simulink model "ZT_VehCtrl_18B"  (R2018b)
settings: Solver=FixedStepAuto  StartTime=0.0  StopTime=inf  FixedStep=0.005  RelTol=1e-3
InitFcn:
  | mbd_mpc_consistency_checks(bdroot(gcs));
undefined symbols (not defined in the file): ANG_DEAD, BMS_NormalPwr, BrkPrsByBrkPct_TB_X, BrkPrsByBrkPct_TB_Y, DELAY_DISCHARGE, DELAY_RCUOFF, DRV_BACKWARD, DRV_BRAKE, DRV_FORWARD, DRV_NEUTRAL, DRV_PARK, DRV_UNPARK, DRV_ZEROTURN, EPB_LOCK, EPB_UNLOCK, ExtraLoadPwr, FanOff, fifo_0_vect, fifo_1_vect, HiFanReq, HV_finished, HV_No_Active, HV_POWER_OFF, HV_POWER_ON, HVDown, HVON, KaTLS_v_DrgUp_X_VehSpd, KeFTM_s_Way1OffDlyTime, KeFTM_TK_Way1CoolLv2OffBatTemp, KeFTM_TK_Way1CoolLv2OffMtrTemp, KeFTM_TK_Way1CoolLv2OnBatTemp, KeFTM_TK_Way1CoolLv2OnMtrTemp, KeFTM_TK_Way1CoolLv3OffBatTemp, KeFTM_TK_Way1CoolLv3OffMtrTemp, KeFTM_TK_Way1CoolLv3OnBatTemp, KeFTM_TK_Way1CoolLv3OnMtrTemp, KeFTM_TK_Way1CoolLv4OffBatTemp, KeFTM_TK_Way1CoolLv4OffMtrTemp, KeFTM_TK_Way1CoolLv4OnBatTemp, KeFTM_TK_Way1CoolLv4OnMtrTemp, Kp1, Kp2, LowFanReq, LQFP, MtrPwrFactor_RCU, MtrPwrHighToMidThd, MtrPwrLowToMidThd, MtrPwrMidToHighThd, MtrPwrMidToLowThd, MtrTrqMax, PCT_DEAD, Precharge, PTO_1000, PTO_540, pts1_fifo_0_vect, pts1_fifo_1_vect, pts2_fifo_0_vect, pts2_fifo_1_vect, pts3_fifo_0_vect, pts3_fifo_1_vect ... (+24)
libraries: mbd_mpc574x_ec_toolbox x124, canmsglib x72, simulink x57
(part 5 of 11)

== system ZT_VehCtrl_18B/SigIn/CAN1/ACU1 ==
  ID : Inport
  Data : Inport  Port=2
  length : Inport  Port=3
  timestamp : Inport  Port=4
  Switch Case : SwitchCase  CaseConditions={hex2dec('0C08A79A')}  ShowDefaultCase=off
  UNPACK : Subsystem  TreatAsAtomicUnit=on
  Message : Outport
  wires:
  Switch Case/1 -> UNPACK/Action
  ID/1 -> UNPACK/1(ID), Switch Case/1
  Data/1 -> UNPACK/2(data)
  timestamp/1 -> UNPACK/4(timestamp)
  length/1 -> UNPACK/3(length)
  UNPACK/1(Message) -> Message/1

== system ZT_VehCtrl_18B/SigIn/CAN1/ACU2 ==
  ID : Inport
  Data : Inport  Port=2
  length : Inport  Port=3
  timestamp : Inport  Port=4
  Switch Case : SwitchCase  CaseConditions={hex2dec('0C09A79B')}  ShowDefaultCase=off
  UNPACK : Subsystem  TreatAsAtomicUnit=on
  Message : Outport
  wires:
  UNPACK/1(Message) -> Message/1
  length/1 -> UNPACK/3(length)
  timestamp/1 -> UNPACK/4(timestamp)
  Data/1 -> UNPACK/2(data)
  ID/1 -> Switch Case/1, UNPACK/1(ID)
  Switch Case/1 -> UNPACK/Action

== system ZT_VehCtrl_18B/SigIn/CAN1/ACU3 ==
  ID : Inport
  Data : Inport  Port=2
  length : Inport  Port=3
  timestamp : Inport  Port=4
  Switch Case : SwitchCase  CaseConditions={hex2dec('0C0AA79D')}  ShowDefaultCase=off
  UNPACK : Subsystem  TreatAsAtomicUnit=on
  Message : Outport
  wires:
  Switch Case/1 -> UNPACK/Action
  ID/1 -> UNPACK/1(ID), Switch Case/1
  Data/1 -> UNPACK/2(data)
  timestamp/1 -> UNPACK/4(timestamp)
  length/1 -> UNPACK/3(length)
  UNPACK/1(Message) -> Message/1

== system ZT_VehCtrl_18B/SigIn/CAN1/HVC1_LV ==
  ID : Inport
  Data : Inport  Port=2
  length : Inport  Port=3
  timestamp : Inport  Port=4
  Switch Case : SwitchCase  CaseConditions={hex2dec('180105A1')}  ShowDefaultCase=off
  UNPACK : Subsystem  TreatAsAtomicUnit=on
  Message : Outport
  wires:
  Switch Case/1 -> UNPACK/Action
  ID/1 -> UNPACK/1(ID), Switch Case/1
  Data/1 -> UNPACK/2(data)
  timestamp/1 -> UNPACK/4(timestamp)
  length/1 -> UNPACK/3(length)
  UNPACK/1(Message) -> Message/1

== system ZT_VehCtrl_18B/SigIn/CAN1/HVC3_Temp ==
  ID : Inport
  Data : Inport  Port=2
  length : Inport  Port=3
  timestamp : Inport  Port=4
  Switch Case : SwitchCase  CaseConditions={hex2dec('180305A1')}  ShowDefaultCase=off
  UNPACK : Subsystem  TreatAsAtomicUnit=on
  Message : Outport
  wires:
  UNPACK/1(Message) -> Message/1
  length/1 -> UNPACK/3(length)
  timestamp/1 -> UNPACK/4(timestamp)
  Data/1 -> UNPACK/2(data)
  ID/1 -> Switch Case/1, UNPACK/1(ID)
  Switch Case/1 -> UNPACK/Action

== system ZT_VehCtrl_18B/SigIn/CAN1/HVC4_RlySt ==
  ID : Inport
  Data : Inport  Port=2
  length : Inport  Port=3
  timestamp : Inport  Port=4
  Switch Case : SwitchCase  CaseConditions={hex2dec('180405A1')}  ShowDefaultCase=off
  UNPACK : Subsystem  TreatAsAtomicUnit=on
  Message : Outport
  wires:
  Switch Case/1 -> UNPACK/Action
  ID/1 -> UNPACK/1(ID), Switch Case/1
  Data/1 -> UNPACK/2(data)
  timestamp/1 -> UNPACK/4(timestamp)
  length/1 -> UNPACK/3(length)
  UNPACK/1(Message) -> Message/1

== system ZT_VehCtrl_18B/SigIn/CAN1/HVC7_HV1 ==
  ID : Inport
  Data : Inport  Port=2
  length : Inport  Port=3
  timestamp : Inport  Port=4
  Switch Case : SwitchCase  CaseConditions={hex2dec('180705A1')}  ShowDefaultCase=off
  UNPACK : Subsystem  TreatAsAtomicUnit=on
  Message : Outport
  wires:
  UNPACK/1(Message) -> Message/1
  length/1 -> UNPACK/3(length)
  timestamp/1 -> UNPACK/4(timestamp)
  Data/1 -> UNPACK/2(data)
  ID/1 -> Switch Case/1, UNPACK/1(ID)
  Switch Case/1 -> UNPACK/Action

== system ZT_VehCtrl_18B/SigIn/CAN1/ISG MCU STATUS 1 ==
  ID : Inport
  Data : Inport  Port=2
  length : Inport  Port=3
  timestamp : Inport  Port=4
  Switch Case : SwitchCase  CaseConditions={hex2dec('CFF0006')}  ShowDefaultCase=off
  UNPACK : Subsystem  TreatAsAtomicUnit=on
  Message : Outport
  wires:
  Switch Case/1 -> UNPACK/Action
  ID/1 -> UNPACK/1(ID), Switch Case/1
  Data/1 -> UNPACK/2(data)
  timestamp/1 -> UNPACK/4(timestamp)
  length/1 -> UNPACK/3(length)
  UNPACK/1(Message) -> Message/1

== system ZT_VehCtrl_18B/SigIn/CAN1/ISG MCU STATUS 2 ==
  ID : Inport
  Data : Inport  Port=2
  length : Inport  Port=3
  timestamp : Inport  Port=4
  Switch Case : SwitchCase  CaseConditions={hex2dec('CFF0106')}  ShowDefaultCase=off
  UNPACK : Subsystem  TreatAsAtomicUnit=on
  Message : Outport
  wires:
  UNPACK/1(Message) -> Message/1
  length/1 -> UNPACK/3(length)
  timestamp/1 -> UNPACK/4(timestamp)
  Data/1 -> UNPACK/2(data)
  ID/1 -> Switch Case/1, UNPACK/1(ID)
  Switch Case/1 -> UNPACK/Action

== system ZT_VehCtrl_18B/SigIn/CAN1/ISG MCU STATUS 3 ==
  ID : Inport
  Data : Inport  Port=2
  length : Inport  Port=3
  timestamp : Inport  Port=4
  Switch Case : SwitchCase  CaseConditions={hex2dec('CFF0206')}  ShowDefaultCase=off
  UNPACK : Subsystem  TreatAsAtomicUnit=on
  Message : Outport
  wires:
  Switch Case/1 -> UNPACK/Action
  ID/1 -> UNPACK/1(ID), Switch Case/1
  Data/1 -> UNPACK/2(data)
  timestamp/1 -> UNPACK/4(timestamp)
  length/1 -> UNPACK/3(length)
  UNPACK/1(Message) -> Message/1

== system ZT_VehCtrl_18B/SigIn/CAN1/MCU1Msg1 ==
  ID : Inport
  Data : Inport  Port=2
  length : Inport  Port=3
  timestamp : Inport  Port=4
  Switch Case : SwitchCase  CaseConditions={hex2dec('1836D0EF')}  ShowDefaultCase=off
  UNPACK : Subsystem  TreatAsAtomicUnit=on
  Message : Outport
  wires:
  UNPACK/1(Message) -> Message/1
  length/1 -> UNPACK/3(length)
  timestamp/1 -> UNPACK/4(timestamp)
  Data/1 -> UNPACK/2(data)
  ID/1 -> Switch Case/1, UNPACK/1(ID)
  Switch Case/1 -> UNPACK/Action

== system ZT_VehCtrl_18B/SigIn/CAN1/MCU1Msg2 ==
  ID : Inport
  Data : Inport  Port=2
  length : Inport  Port=3
  timestamp : Inport  Port=4
  Switch Case : SwitchCase  CaseConditions={hex2dec('1837D0EF')}  ShowDefaultCase=off
  UNPACK : Subsystem  TreatAsAtomicUnit=on
  Message : Outport
  wires:
  Switch Case/1 -> UNPACK/Action
  ID/1 -> UNPACK/1(ID), Switch Case/1
  Data/1 -> UNPACK/2(data)
  timestamp/1 -> UNPACK/4(timestamp)
  length/1 -> UNPACK/3(length)
  UNPACK/1(Message) -> Message/1

== system ZT_VehCtrl_18B/SigIn/CAN1/MCU1Msg3 ==
  ID : Inport
  Data : Inport  Port=2
  length : Inport  Port=3
  timestamp : Inport  Port=4
  Switch Case : SwitchCase  CaseConditions={hex2dec('1838D0EF')}  ShowDefaultCase=off
  UNPACK : Subsystem  TreatAsAtomicUnit=on
  Message : Outport
  wires:
  UNPACK/1(Message) -> Message/1
  length/1 -> UNPACK/3(length)
  timestamp/1 -> UNPACK/4(timestamp)
  Data/1 -> UNPACK/2(data)
  ID/1 -> Switch Case/1, UNPACK/1(ID)
  Switch Case/1 -> UNPACK/Action

== system ZT_VehCtrl_18B/SigIn/CAN1/MCU2Msg1 ==
  ID : Inport
  Data : Inport  Port=2
  length : Inport  Port=3
  timestamp : Inport  Port=4
  Switch Case : SwitchCase  CaseConditions={hex2dec('1836D0F1')}  ShowDefaultCase=off
  UNPACK : Subsystem  TreatAsAtomicUnit=on
  Message : Outport
  wires:
  Switch Case/1 -> UNPACK/Action
  ID/1 -> UNPACK/1(ID), Switch Case/1
  Data/1 -> UNPACK/2(data)
  timestamp/1 -> UNPACK/4(timestamp)
  length/1 -> UNPACK/3(length)
  UNPACK/1(Message) -> Message/1

== system ZT_VehCtrl_18B/SigIn/CAN1/MCU2Msg2 ==
  ID : Inport
  Data : Inport  Port=2
  length : Inport  Port=3
  timestamp : Inport  Port=4
  Switch Case : SwitchCase  CaseConditions={hex2dec('1837D0F1')}  ShowDefaultCase=off
  UNPACK : Subsystem  TreatAsAtomicUnit=on
  Message : Outport
  wires:
  UNPACK/1(Message) -> Message/1
  length/1 -> UNPACK/3(length)
  timestamp/1 -> UNPACK/4(timestamp)
  Data/1 -> UNPACK/2(data)
  ID/1 -> Switch Case/1, UNPACK/1(ID)
  Switch Case/1 -> UNPACK/Action

== system ZT_VehCtrl_18B/SigIn/CAN1/MCU2Msg3 ==
  ID : Inport
  Data : Inport  Port=2
  length : Inport  Port=3
  timestamp : Inport  Port=4
  Switch Case : SwitchCase  CaseConditions={hex2dec('1838D0F1')}  ShowDefaultCase=off
  UNPACK : Subsystem  TreatAsAtomicUnit=on
  Message : Outport
  wires:
  Switch Case/1 -> UNPACK/Action
  ID/1 -> UNPACK/1(ID), Switch Case/1
  Data/1 -> UNPACK/2(data)
  timestamp/1 -> UNPACK/4(timestamp)
  length/1 -> UNPACK/3(length)
  UNPACK/1(Message) -> Message/1

== system ZT_VehCtrl_18B/SigIn/CAN1/PDU_RelaySts ==
  ID : Inport
  Data : Inport  Port=2
  length : Inport  Port=3
  timestamp : Inport  Port=4
  Switch Case : SwitchCase  CaseConditions={hex2dec('18FF2BC8')}  ShowDefaultCase=off
  UNPACK : Subsystem  TreatAsAtomicUnit=on
  Message : Outport
  wires:
  UNPACK/1(Message) -> Message/1
  length/1 -> UNPACK/3(length)
  timestamp/1 -> UNPACK/4(timestamp)
  Data/1 -> UNPACK/2(data)
  ID/1 -> Switch Case/1, UNPACK/1(ID)
  Switch Case/1 -> UNPACK/Action

== system ZT_VehCtrl_18B/SigIn/CAN1/TM MCU STATUS 1 ==
  ID : Inport
  Data : Inport  Port=2
  length : Inport  Port=3
  timestamp : Inport  Port=4
  Switch Case : SwitchCase  CaseConditions={hex2dec('CFF0005')}  ShowDefaultCase=off
  UNPACK : Subsystem  TreatAsAtomicUnit=on
  Message : Outport
  wires:
  UNPACK/1(Message) -> Message/1
  length/1 -> UNPACK/3(length)
  timestamp/1 -> UNPACK/4(timestamp)
  Data/1 -> UNPACK/2(data)
  ID/1 -> Switch Case/1, UNPACK/1(ID)
  Switch Case/1 -> UNPACK/Action

== system ZT_VehCtrl_18B/SigIn/CAN1/TM MCU STATUS 2 ==
  ID : Inport
  Data : Inport  Port=2
  length : Inport  Port=3
  timestamp : Inport  Port=4
  Switch Case : SwitchCase  CaseConditions={hex2dec('CFF0105')}  ShowDefaultCase=off
  UNPACK : Subsystem  TreatAsAtomicUnit=on
  Message : Outport
  wires:
  Switch Case/1 -> UNPACK/Action
  ID/1 -> UNPACK/1(ID), Switch Case/1
  Data/1 -> UNPACK/2(data)
  timestamp/1 -> UNPACK/4(timestamp)
  length/1 -> UNPACK/3(length)
  UNPACK/1(Message) -> Message/1

== system ZT_VehCtrl_18B/SigIn/CAN1/TM MCU STATUS 3 ==
  ID : Inport
  Data : Inport  Port=2
  length : Inport  Port=3
  timestamp : Inport  Port=4
  Switch Case : SwitchCase  CaseConditions={hex2dec('CFF0205')}  ShowDefaultCase=off
  UNPACK : Subsystem  TreatAsAtomicUnit=on
  Message : Outport
  wires:
  UNPACK/1(Message) -> Message/1
  length/1 -> UNPACK/3(length)
  timestamp/1 -> UNPACK/4(timestamp)
  Data/1 -> UNPACK/2(data)
  ID/1 -> Switch Case/1, UNPACK/1(ID)
  Switch Case/1 -> UNPACK/Action

== system ZT_VehCtrl_18B/SigIn/CAN1/TWV  ==
  ID : Inport
  Data : Inport  Port=2
  length : Inport  Port=3
  timestamp : Inport  Port=4
  Switch Case : SwitchCase  CaseConditions={hex2dec('18FF243B')}  ShowDefaultCase=off
  UNPACK : Subsystem  TreatAsAtomicUnit=on
  Message : Outport
  wires:
  Switch Case/1 -> UNPACK/Action
  ID/1 -> UNPACK/1(ID), Switch Case/1
  Data/1 -> UNPACK/2(data)
  timestamp/1 -> UNPACK/4(timestamp)
  length/1 -> UNPACK/3(length)
  UNPACK/1(Message) -> Message/1

== system ZT_VehCtrl_18B/SigIn/DI/DI_31_32_33_34 ==
  note: DI PWM PULLUP
  note: DI PWM PULLDOWN
  DI31 : mbd_mpc574x_ec_toolbox/GPIO Blocks/Digital_Input  gpio_pin=PTF0: [SIUL2_GPIO80 | General Purpose IO PF[0]]  pull_resistor=None
  DI32 : mbd_mpc574x_ec_toolbox/GPIO Blocks/Digital_Input  gpio_pin=PTD1: [SIUL2_GPIO49 | General Purpose IO PD[1]]  pull_resistor=None
  DI33 : mbd_mpc574x_ec_toolbox/GPIO Blocks/Digital_Input  gpio_pin=PTD2: [SIUL2_GPIO50 | General Purpose IO PD[2]]  pull_resistor=None
  DI34 : mbd_mpc574x_ec_toolbox/GPIO Blocks/Digital_Input  gpio_pin=PTC13: [SIUL2_GPIO45 | General Purpose IO PC[13]]  pull_resistor=None
  Data Store Write14 : DataStoreWrite  DataStoreName=DI31
  Data Store Write15 : DataStoreWrite  DataStoreName=DI32
  Data Store Write16 : DataStoreWrite  DataStoreName=DI33
  Data Store Write17 : DataStoreWrite  DataStoreName=DI34
  wires:
  DI34/1 -> Data Store Write17/1
  DI33/1 -> Data Store Write16/1
  DI32/1 -> Data Store Write15/1
  DI31/1 -> Data Store Write14/1

== system ZT_VehCtrl_18B/SigIn/PWM/PWM_PTS1 ==
  Add : Sum  Inputs=+-  AccumDataTypeStr=single
  Add1 : Sum  Inputs=+-  AccumDataTypeStr=single
  Data Store Memory : DataStoreMemory  DataStoreName=pts1_pwm_cnt  ReadBeforeWriteMsg=warning  WriteAfterWriteMsg=warning  WriteAfterReadMsg=warning  ShowAdditionalParam=off  OutDataTypeStr=uint8
  Data Store Memory2 : DataStoreMemory  DataStoreName=pts1_fifo_1_vect  ReadBeforeWriteMsg=warning  WriteAfterWriteMsg=warning  WriteAfterReadMsg=warning  InitialValue=[0 0 0 0 0 0 0 0]  ShowAdditionalParam=off  OutDataTypeStr=uint16
  Data Store Memory4 : DataStoreMemory  DataStoreName=pts1_fifo_0_vect  ReadBeforeWriteMsg=warning  WriteAfterWriteMsg=warning  WriteAfterReadMsg=warning  InitialValue=[0 0 0 0 0 0 0 0]  ShowAdditionalParam=off  OutDataTypeStr=uint16
  Data Store Read : DataStoreRead  DataStoreName=pts1_fifo_0_vect  DataStoreElements=pts1_fifo_0_vect(2)#pts1_fifo_0_vect(1)
  Data Store Read1 : DataStoreRead  DataStoreName=pts1_fifo_1_vect  DataStoreElements=pts1_fifo_1_vect(1)
  Data Store Read2 : DataStoreRead  DataStoreName=pts1_fifo_0_vect  DataStoreElements=pts1_fifo_0_vect(1)
  Data Store Write3 : DataStoreWrite  DataStoreName=pts1_fifo_0_vect
  Data Store Write5 : DataStoreWrite  DataStoreName=pts1_fifo_1_vect
  Divide : Product  Inputs=*/  OutDataTypeStr=single
  Divide1 : Product  Inputs=*//
  Freq_MC : Constant  Value=80000000  OutDataTypeStr=single
  Prescaler : Constant  Value=32  OutDataTypeStr=single
  Subsystem : Subsystem
  Subsystem_capture : Subsystem
  Terminator1 : Terminator
  Terminator2 : Terminator
  eTimer_ISR : mbd_mpc574x_ec_toolbox/Motor Control Blocks/eTIMER Blocks/eTimer_ISR_Handler  etimerModule=1  etimerInterrupt=Channel Interrupt  etimerChannel=2  etimerIsrPriority=14
      settings: SourceProductName=NXP Model-Based Design Toolbox for MPC57xx MCUs
  DC : Outport
  freq : Outport  Port=2
  wires:
  eTimer_ISR/2 -> Subsystem_capture/1(In1)
  Subsystem_capture/1(Out1) -> Terminator1/1
  Subsystem_capture/3(Out3) -> Terminator2/1
  Subsystem_capture/4(Out4) -> Data Store Write5/1
  Subsystem_capture/2(Out2) -> Data Store Write3/1
  eTimer_ISR/1 -> Subsystem_capture/Trigger
  Prescaler/1 -> Divide1/2
  Add/1 -> Divide/2, Divide1/3
  Data Store Read1/1 -> Add1/1
  Data Store Read/2 -> Add/2
  Freq_MC/1 -> Divide1/1
  Add1/1 -> Divide/1
  Data Store Read2/1 -> Add1/2
  Divide1/1 -> freq/1
  Data Store Read/1 -> Add/1
  Divide/1 -> Subsystem/1(In1)
  Subsystem/1(Out1) -> DC/1

== system ZT_VehCtrl_18B/SigIn/PWM/PWM_PTS2 ==
  Add : Sum  Inputs=+-  AccumDataTypeStr=single
  Add1 : Sum  Inputs=+-  AccumDataTypeStr=single
  Data Store Memory : DataStoreMemory  DataStoreName=pts2_pwm_cnt  ReadBeforeWriteMsg=warning  WriteAfterWriteMsg=warning  WriteAfterReadMsg=warning  ShowAdditionalParam=off  OutDataTypeStr=uint8
  Data Store Memory2 : DataStoreMemory  DataStoreName=pts2_fifo_1_vect  ReadBeforeWriteMsg=warning  WriteAfterWriteMsg=warning  WriteAfterReadMsg=warning  InitialValue=[0 0 0 0 0 0 0 0]  ShowAdditionalParam=off  OutDataTypeStr=uint16
  Data Store Memory4 : DataStoreMemory  DataStoreName=pts2_fifo_0_vect  ReadBeforeWriteMsg=warning  WriteAfterWriteMsg=warning  WriteAfterReadMsg=warning  InitialValue=[0 0 0 0 0 0 0 0]  ShowAdditionalParam=off  OutDataTypeStr=uint16
  Data Store Read : DataStoreRead  DataStoreName=pts2_fifo_0_vect  DataStoreElements=pts2_fifo_0_vect(2)#pts2_fifo_0_vect(1)
  Data Store Read1 : DataStoreRead  DataStoreName=pts2_fifo_1_vect  DataStoreElements=pts2_fifo_1_vect(1)
  Data Store Read2 : DataStoreRead  DataStoreName=pts2_fifo_0_vect  DataStoreElements=pts2_fifo_0_vect(1)
  Data Store Write3 : DataStoreWrite  DataStoreName=pts2_fifo_0_vect
  Data Store Write5 : DataStoreWrite  DataStoreName=pts2_fifo_1_vect
  Divide : Product  Inputs=*/  OutDataTypeStr=single
  Divide1 : Product  Inputs=*//
  Freq_MC : Constant  Value=80000000  OutDataTypeStr=single
  Prescaler : Constant  Value=32  OutDataTypeStr=single
  Subsystem : Subsystem
  Subsystem_capture : Subsystem
  Terminator1 : Terminator
  Terminator2 : Terminator
  eTimer_ISR : mbd_mpc574x_ec_toolbox/Motor Control Blocks/eTIMER Blocks/eTimer_ISR_Handler  etimerModule=1  etimerInterrupt=Channel Interrupt  etimerChannel=3  etimerIsrPriority=14
      settings: SourceProductName=NXP Model-Based Design Toolbox for MPC57xx MCUs
  DC : Outport
  freq : Outport  Port=2
  wires:
  Subsystem/1(Out1) -> DC/1
  Divide/1 -> Subsystem/1(In1)
  Data Store Read/1 -> Add/1
  Divide1/1 -> freq/1
  Data Store Read2/1 -> Add1/2
  Add1/1 -> Divide/1
  Freq_MC/1 -> Divide1/1
  Data Store Read/2 -> Add/2
  Data Store Read1/1 -> Add1/1
  Add/1 -> Divide1/3, Divide/2
  Prescaler/1 -> Divide1/2
  eTimer_ISR/1 -> Subsystem_capture/Trigger
  Subsystem_capture/2(Out2) -> Data Store Write3/1
  Subsystem_capture/4(Out4) -> Data Store Write5/1
  Subsystem_capture/3(Out3) -> Terminator2/1
  Subsystem_capture/1(Out1) -> Terminator1/1
  eTimer_ISR/2 -> Subsystem_capture/1(In1)

== system ZT_VehCtrl_18B/SigIn/PWM/PWM_PTS3 ==
  Add : Sum  Inputs=+-  AccumDataTypeStr=single
  Add1 : Sum  Inputs=+-  AccumDataTypeStr=single
  Data Store Memory : DataStoreMemory  DataStoreName=pts3_pwm_cnt  ReadBeforeWriteMsg=warning  WriteAfterWriteMsg=warning  WriteAfterReadMsg=warning  ShowAdditionalParam=off  OutDataTypeStr=uint8
  Data Store Memory2 : DataStoreMemory  DataStoreName=pts3_fifo_1_vect  ReadBeforeWriteMsg=warning  WriteAfterWriteMsg=warning  WriteAfterReadMsg=warning  InitialValue=[0 0 0 0 0 0 0 0]  ShowAdditionalParam=off  OutDataTypeStr=uint16
  Data Store Memory4 : DataStoreMemory  DataStoreName=pts3_fifo_0_vect  ReadBeforeWriteMsg=warning  WriteAfterWriteMsg=warning  WriteAfterReadMsg=warning  InitialValue=[0 0 0 0 0 0 0 0]  ShowAdditionalParam=off  OutDataTypeStr=uint16
  Data Store Read : DataStoreRead  DataStoreName=pts3_fifo_0_vect  DataStoreElements=pts3_fifo_0_vect(2)#pts3_fifo_0_vect(1)
  Data Store Read1 : DataStoreRead  DataStoreName=pts3_fifo_1_vect  DataStoreElements=pts3_fifo_1_vect(1)
  Data Store Read2 : DataStoreRead  DataStoreName=pts3_fifo_0_vect  DataStoreElements=pts3_fifo_0_vect(1)
  Data Store Write3 : DataStoreWrite  DataStoreName=pts3_fifo_0_vect
  Data Store Write5 : DataStoreWrite  DataStoreName=pts3_fifo_1_vect
  Divide : Product  Inputs=*/  OutDataTypeStr=single
  Divide1 : Product  Inputs=*//
  Freq_MC : Constant  Value=80000000  OutDataTypeStr=single
  Prescaler : Constant  Value=32  OutDataTypeStr=single
  Subsystem : Subsystem
  Subsystem_capture : Subsystem
  Terminator1 : Terminator
  Terminator2 : Terminator
  eTimer_ISR : mbd_mpc574x_ec_toolbox/Motor Control Blocks/eTIMER Blocks/eTimer_ISR_Handler  etimerModule=1  etimerInterrupt=Channel Interrupt  etimerChannel=1  etimerIsrPriority=14
      settings: SourceProductName=NXP Model-Based Design Toolbox for MPC57xx MCUs
  DC : Outport
  freq : Outport  Port=2
  wires:
  eTimer_ISR/2 -> Subsystem_capture/1(In1)
  Subsystem_capture/1(Out1) -> Terminator1/1
  Subsystem_capture/3(Out3) -> Terminator2/1
  Subsystem_capture/4(Out4) -> Data Store Write5/1
  Subsystem_capture/2(Out2) -> Data Store Write3/1
  eTimer_ISR/1 -> Subsystem_capture/Trigger
  Prescaler/1 -> Divide1/2
  Add/1 -> Divide/2, Divide1/3
  Data Store Read1/1 -> Add1/1
  Data Store Read/2 -> Add/2
  Freq_MC/1 -> Divide1/1
  Add1/1 -> Divide/1
  Data Store Read2/1 -> Add1/2
  Divide1/1 -> freq/1
  Data Store Read/1 -> Add/1
  Divide/1 -> Subsystem/1(In1)
  Subsystem/1(Out1) -> DC/1

== system ZT_VehCtrl_18B/SigIn/PWM/PWM_PTS4 ==
  Add : Sum  Inputs=+-  AccumDataTypeStr=single
  Add1 : Sum  Inputs=+-  AccumDataTypeStr=single
  Data Store Memory : DataStoreMemory  DataStoreName=pts4_pwm_cnt  ReadBeforeWriteMsg=warning  WriteAfterWriteMsg=warning  WriteAfterReadMsg=warning  ShowAdditionalParam=off  OutDataTypeStr=uint8
  Data Store Memory2 : DataStoreMemory  DataStoreName=pts4_fifo_1_vect  ReadBeforeWriteMsg=warning  WriteAfterWriteMsg=warning  WriteAfterReadMsg=warning  InitialValue=[0 0 0 0 0 0 0 0]  ShowAdditionalParam=off  OutDataTypeStr=uint16
  Data Store Memory4 : DataStoreMemory  DataStoreName=pts4_fifo_0_vect  ReadBeforeWriteMsg=warning  WriteAfterWriteMsg=warning  WriteAfterReadMsg=warning  InitialValue=[0 0 0 0 0 0 0 0]  ShowAdditionalParam=off  OutDataTypeStr=uint16
  Data Store Read : DataStoreRead  DataStoreName=pts4_fifo_0_vect  DataStoreElements=pts4_fifo_0_vect(2)#pts4_fifo_0_vect(1)
  Data Store Read1 : DataStoreRead  DataStoreName=pts4_fifo_1_vect  DataStoreElements=pts4_fifo_1_vect(1)
  Data Store Read2 : DataStoreRead  DataStoreName=pts4_fifo_0_vect  DataStoreElements=pts4_fifo_0_vect(1)
  Data Store Write3 : DataStoreWrite  DataStoreName=pts4_fifo_0_vect
  Data Store Write5 : DataStoreWrite  DataStoreName=pts4_fifo_1_vect
  Divide : Product  Inputs=*/  OutDataTypeStr=single
  Divide1 : Product  Inputs=*//
  Freq_MC : Constant  Value=80000000  OutDataTypeStr=single
  Prescaler : Constant  Value=32  OutDataTypeStr=single
  Subsystem : Subsystem
  Subsystem_capture : Subsystem
  Terminator1 : Terminator
  Terminator2 : Terminator
  eTimer_ISR : mbd_mpc574x_ec_toolbox/Motor Control Blocks/eTIMER Blocks/eTimer_ISR_Handler  etimerModule=0  etimerInterrupt=Channel Interrupt  etimerChannel=2  etimerIsrPriority=14
      settings: SourceProductName=NXP Model-Based Design Toolbox for MPC57xx MCUs
  DC : Outport
  freq : Outport  Port=2
  wires:
  Subsystem/1(Out1) -> DC/1
  Divide/1 -> Subsystem/1(In1)
  Data Store Read/1 -> Add/1
  Divide1/1 -> freq/1
  Data Store Read2/1 -> Add1/2
  Add1/1 -> Divide/1
  Freq_MC/1 -> Divide1/1
  Data Store Read/2 -> Add/2
  Data Store Read1/1 -> Add1/1
  Add/1 -> Divide1/3, Divide/2
  Prescaler/1 -> Divide1/2
  eTimer_ISR/1 -> Subsystem_capture/Trigger
  Subsystem_capture/2(Out2) -> Data Store Write3/1
  Subsystem_capture/4(Out4) -> Data Store Write5/1
  Subsystem_capture/3(Out3) -> Terminator2/1
  Subsystem_capture/1(Out1) -> Terminator1/1
  eTimer_ISR/2 -> Subsystem_capture/1(In1)

== system ZT_VehCtrl_18B/SigIn/PWM/Subsystem ==
  Data Store Memory1 : DataStoreMemory  DataStoreName=fifo_1_value  ReadBeforeWriteMsg=warning  WriteAfterWriteMsg=warning  WriteAfterReadMsg=warning  VectorParams1D=off  ShowAdditionalParam=off  OutDataTypeStr=uint16
  Data Store Memory3 : DataStoreMemory  DataStoreName=fifo_0_value  ReadBeforeWriteMsg=warning  WriteAfterWriteMsg=warning  WriteAfterReadMsg=warning  VectorParams1D=off  ShowAdditionalParam=off  OutDataTypeStr=uint16
  Data Store Memory5 : DataStoreMemory  DataStoreName=frequency  ReadBeforeWriteMsg=warning  WriteAfterWriteMsg=warning  WriteAfterReadMsg=warning  VectorParams1D=off  ShowAdditionalParam=off  OutDataTypeStr=single
  Data Store Memory6 : DataStoreMemory  DataStoreName=duty_cycle  ReadBeforeWriteMsg=warning  WriteAfterWriteMsg=warning  WriteAfterReadMsg=warning  VectorParams1D=off  ShowAdditionalParam=off  OutDataTypeStr=single
  Data Store Write10 : DataStoreWrite  DataStoreName=fifo_0_vect
  Data Store Write11 : DataStoreWrite  DataStoreName=fifo_1_value
  Data Store Write12 : DataStoreWrite  DataStoreName=fifo_1_vect
  Data Store Write13 : DataStoreWrite  DataStoreName=duty_cycle
  Data Store Write8 : DataStoreWrite  DataStoreName=frequency
  Data Store Write9 : DataStoreWrite  DataStoreName=fifo_0_value
  Frequency_DutyCycle_Computation : Subsystem
  eTimer Configuration and Signal Measurements : Subsystem
  wires:
  eTimer Configuration and Signal Measurements/4(Out4) -> Data Store Write12/1
  eTimer Configuration and Signal Measurements/2(Out2) -> Data Store Write10/1
  eTimer Configuration and Signal Measurements/3(Out3) -> Data Store Write11/1
  eTimer Configuration and Signal Measurements/1(Out1) -> Data Store Write9/1
  Frequency_DutyCycle_Computation/2(Out2) -> Data Store Write8/1
  Frequency_DutyCycle_Computation/1(Out1) -> Data Store Write13/1

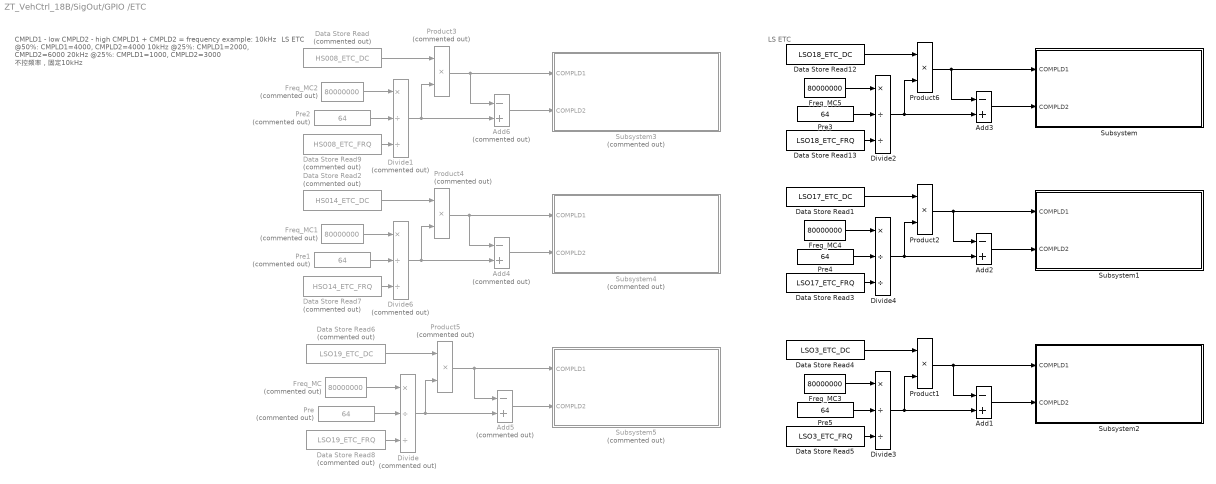
== system ZT_VehCtrl_18B/SigOut/GPIO /ETC ==
  note: CMPLD1 - low
      | CMPLD2 - high
      | CMPLD1 + CMPLD2 = frequency
      | example:
      | 10kHz @50%: CMPLD1=4000, CMPLD2=4000
      | 10kHz @25%: CMPLD1=2000, CMPLD2=6000
      | 20kHz @25%: CMPLD1=1000, CMPLD2=3000
      |
      | 不控频率，固定10kHz
  note: LS ETC
  note: LS ETC
  Add1 : Sum  Inputs=-+
  Add2 : Sum  Inputs=-+
  Add3 : Sum  Inputs=-+
  Add4 : Sum  Commented=on  Inputs=-+
  Add5 : Sum  Commented=on  Inputs=-+
  Add6 : Sum  Commented=on  Inputs=-+
  Data Store Read : DataStoreRead  Commented=on  DataStoreName=HS008_ETC_DC
  Data Store Read1 : DataStoreRead  DataStoreName=LSO17_ETC_DC
  Data Store Read12 : DataStoreRead  DataStoreName=LSO18_ETC_DC
  Data Store Read13 : DataStoreRead  DataStoreName=LSO18_ETC_FRQ
  Data Store Read2 : DataStoreRead  Commented=on  DataStoreName=HS014_ETC_DC
  Data Store Read3 : DataStoreRead  DataStoreName=LSO17_ETC_FRQ
  Data Store Read4 : DataStoreRead  DataStoreName=LSO3_ETC_DC
  Data Store Read5 : DataStoreRead  DataStoreName=LSO3_ETC_FRQ
  Data Store Read6 : DataStoreRead  Commented=on  DataStoreName=LSO19_ETC_DC
  Data Store Read7 : DataStoreRead  Commented=on  DataStoreName=HSO14_ETC_FRQ
  Data Store Read8 : DataStoreRead  Commented=on  DataStoreName=LSO19_ETC_FRQ
  Data Store Read9 : DataStoreRead  Commented=on  DataStoreName=HS008_ETC_FRQ
  Divide : Product  Commented=on  Inputs=*//
  Divide1 : Product  Commented=on  Inputs=*//
  Divide2 : Product  Inputs=*//
  Divide3 : Product  Inputs=*//
  Divide4 : Product  Inputs=*//
  Divide6 : Product  Commented=on  Inputs=*//
  Freq_MC : Constant  Commented=on  Value=80000000  OutDataTypeStr=single
  Freq_MC1 : Constant  Commented=on  Value=80000000  OutDataTypeStr=single
  Freq_MC2 : Constant  Commented=on  Value=80000000  OutDataTypeStr=single
  Freq_MC3 : Constant  Value=80000000  OutDataTypeStr=single
  Freq_MC4 : Constant  Value=80000000  OutDataTypeStr=single
  Freq_MC5 : Constant  Value=80000000  OutDataTypeStr=single
  Pre : Constant  Commented=on  Value=64
  Pre1 : Constant  Commented=on  Value=64
  Pre2 : Constant  Commented=on  Value=64
  Pre3 : Constant  Value=64
  Pre4 : Constant  Value=64
  Pre5 : Constant  Value=64
  Product1 : Product
  Product2 : Product
  Product3 : Product  Commented=on
  Product4 : Product  Commented=on
  Product5 : Product  Commented=on
  Product6 : Product
  Subsystem : Subsystem
  Subsystem1 : Subsystem
  Subsystem2 : Subsystem
  Subsystem3 : Subsystem  Commented=on
  Subsystem4 : Subsystem  Commented=on
  Subsystem5 : Subsystem  Commented=on
  wires:
  Data Store Read6/1 -> Product5/1
  Product5/1 -> Add5/1, Subsystem5/1(COMPLD1)
  Add5/1 -> Subsystem5/2(COMPLD2)
  Add4/1 -> Subsystem4/2(COMPLD2)
  Data Store Read8/1 -> Divide/3
  Data Store Read2/1 -> Product4/1
  Freq_MC/1 -> Divide/1
  Divide/1 -> Product5/2, Add5/2
  Divide6/1 -> Product4/2, Add4/2
  Freq_MC1/1 -> Divide6/1
  Data Store Read7/1 -> Divide6/3
  Product4/1 -> Add4/1, Subsystem4/1(COMPLD1)
  Divide1/1 -> Product3/2, Add6/2
  Freq_MC2/1 -> Divide1/1
  Data Store Read9/1 -> Divide1/3
  Product3/1 -> Add6/1, Subsystem3/1(COMPLD1)
  Data Store Read/1 -> Product3/1
  Add6/1 -> Subsystem3/2(COMPLD2)
  Divide3/1 -> Product1/2, Add1/2
  Freq_MC3/1 -> Divide3/1
  Data Store Read5/1 -> Divide3/3
  Product1/1 -> Add1/1, Subsystem2/1(COMPLD1)
  Divide4/1 -> Product2/2, Add2/2
  Freq_MC4/1 -> Divide4/1
  Data Store Read3/1 -> Divide4/3
  Product2/1 -> Add2/1, Subsystem1/1(COMPLD1)
  Divide2/1 -> Product6/2, Add3/2
  Freq_MC5/1 -> Divide2/1
  Data Store Read13/1 -> Divide2/3
  Product6/1 -> Add3/1, Subsystem/1(COMPLD1)
  Data Store Read1/1 -> Product2/1
  Data Store Read4/1 -> Product1/1
  Data Store Read12/1 -> Product6/1
  Add1/1 -> Subsystem2/2(COMPLD2)
  Add2/1 -> Subsystem1/2(COMPLD2)
  Add3/1 -> Subsystem/2(COMPLD2)
  Pre/1 -> Divide/2
  Pre1/1 -> Divide6/2
  Pre2/1 -> Divide1/2
  Pre3/1 -> Divide2/2
  Pre4/1 -> Divide4/2
  Pre5/1 -> Divide3/2

== system ZT_VehCtrl_18B/SigOut/GPIO /HS ==
  note: 3A/5A
  note: 1A/3A
  note: 0.5A/1A
  Data Store Read : DataStoreRead  DataStoreName=HS001
  Data Store Read2 : DataStoreRead  DataStoreName=HS007
  Data Store Read4 : DataStoreRead  DataStoreName=HS002
  Data Store Read5 : DataStoreRead  DataStoreName=HS003
  Data Store Read6 : DataStoreRead  DataStoreName=HS004
  Data Store Read7 : DataStoreRead  DataStoreName=HS005
  Data Store Read9 : DataStoreRead  DataStoreName=HS010
  HS001 : mbd_mpc574x_ec_toolbox/GPIO Blocks/Digital_Output  Priority=1  gpio_pin=PTF5: [SIUL2_GPIO85 | General Purpose IO PF[5]]  gpio_drive_strength=Disabled
  "HS002 " : mbd_mpc574x_ec_toolbox/GPIO Blocks/Digital_Output  Priority=1  gpio_pin=PTF4: [SIUL2_GPIO84 | General Purpose IO PF[4]]  gpio_drive_strength=Disabled
  HS003 : mbd_mpc574x_ec_toolbox/GPIO Blocks/Digital_Output  Priority=1  gpio_pin=PTF3: [SIUL2_GPIO83 | General Purpose IO PF[3]]  gpio_drive_strength=Disabled
  HS004 : mbd_mpc574x_ec_toolbox/GPIO Blocks/Digital_Output  Priority=1  gpio_pin=PTB6: [SIUL2_GPIO22 | General Purpose IO PB[6]]  gpio_drive_strength=Disabled
  HS005 : mbd_mpc574x_ec_toolbox/GPIO Blocks/Digital_Output  Priority=1  gpio_pin=PTA12: [SIUL2_GPIO12 | General Purpose IO PA[12]]  gpio_drive_strength=Disabled
  HS007 : mbd_mpc574x_ec_toolbox/GPIO Blocks/Digital_Output  Priority=1  gpio_pin=PTF7: [SIUL2_GPIO87 | General Purpose IO PF[7]]  gpio_drive_strength=Disabled
  HS010 : mbd_mpc574x_ec_toolbox/GPIO Blocks/Digital_Output  Priority=1  gpio_pin=PTF9: [SIUL2_GPIO89 | General Purpose IO PF[9]]  gpio_drive_strength=Disabled
  wires:
  Data Store Read/1 -> HS001/1
  Data Store Read5/1 -> HS003/1
  Data Store Read4/1 -> "HS002 "/1
  Data Store Read6/1 -> HS004/1
  Data Store Read7/1 -> HS005/1
  Data Store Read2/1 -> HS007/1
  Data Store Read9/1 -> HS010/1

== system ZT_VehCtrl_18B/SigOut/GPIO /PWM_OUT ==
  note: LS PWM
  note: HS PWM
  note: Example
  Data Store Read10 : DataStoreRead  DataStoreName=HSO14_PWM_DC
  Data Store Read11 : DataStoreRead  DataStoreName=HSO14_PWM_FRQ
  Data Store Read14 : DataStoreRead  DataStoreName=LSO19_PWM_DC
  Data Store Read15 : DataStoreRead  DataStoreName=LSO19_PWM_FRQ
  Data Store Read2 : DataStoreRead  DataStoreName=HSO08_PWM_DC
  Data Store Read9 : DataStoreRead  DataStoreName=HSO08_PWM_FRQ
  FreqCMD : Stateflow chart  Priority=0  Commented=on  TreatAsAtomicUnit=on
  PWM Configuration and Frequency Update : Subsystem  Commented=on
  PWM Configuration and Frequency Update1 : Subsystem
  PWM Configuration and Frequency Update4 : Subsystem
  wires:
  FreqCMD/1(freq) -> PWM Configuration and Frequency Update/1(In1)
  FreqCMD/2(dc) -> PWM Configuration and Frequency Update/2(In2)
  Data Store Read9/1 -> PWM Configuration and Frequency Update1/2(Fre A)
  Data Store Read2/1 -> PWM Configuration and Frequency Update1/1(PWM A)
  Data Store Read14/1 -> PWM Configuration and Frequency Update4/1(PWM A)
  Data Store Read10/1 -> PWM Configuration and Frequency Update1/3(PWM B)
  Data Store Read11/1 -> PWM Configuration and Frequency Update1/4(Fre B)
  Data Store Read15/1 -> PWM Configuration and Frequency Update4/2(Fre)

== system ZT_VehCtrl_18B/SigOut/GPIO /SPI0: LS09_14_15_16_1_2_11_4 ==
  note: 不要开，会重置SPI的初始化设置
  Compare To Constant : simulink/Logic and Bit Operations/Compare To Constant  relop===  const=2  OutDataTypeStr=boolean
  Constant : Constant  OutDataTypeStr=boolean
  Constant1 : Constant  OutDataTypeStr=boolean
  Constant2 : Constant  OutDataTypeStr=boolean
  Data Store Read : DataStoreRead  DataStoreName=VCU_Mode
  Data Store Read1 : DataStoreRead  DataStoreName=SPI0_CS
  LS_CTRL : Subsystem
  LS_CTRL1 : Subsystem
  LS_EN : mbd_mpc574x_ec_toolbox/GPIO Blocks/Digital_Output  Priority=1  gpio_pin=PTA2: [SIUL2_GPIO2 | General Purpose IO PA[2]]  gpio_drive_strength=Disabled
  LS_rst1 : mbd_mpc574x_ec_toolbox/GPIO Blocks/Digital_Output  Priority=1  gpio_pin=PTC10: [SIUL2_GPIO42 | General Purpose IO PC[10]]  gpio_drive_strength=Disabled
  LS_rst2 : mbd_mpc574x_ec_toolbox/GPIO Blocks/Digital_Output  Priority=1  gpio_pin=PTA1: [SIUL2_GPIO1 | General Purpose IO PA[1]]  gpio_drive_strength=Disabled
  Logical Operator : Logic  AllPortsSameDT=off  OutDataTypeStr=boolean
  Logical Operator1 : Logic  Operator=NOT  AllPortsSameDT=off  OutDataTypeStr=boolean
  wires:
  Constant1/1 -> LS_rst2/1
  Constant/1 -> LS_EN/1
  Constant2/1 -> LS_rst1/1
  Data Store Read/1 -> Compare To Constant/1
  Compare To Constant/1 -> Logical Operator/1
  Data Store Read1/1 -> Logical Operator/2
  Logical Operator/1 -> LS_CTRL1/Enable, Logical Operator1/1
  Logical Operator1/1 -> LS_CTRL/Enable

== system ZT_VehCtrl_18B/SigOut/GPIO /SPI3: LS03_06_07_08_10_12_13_17_18_19 ==
  Compare To Constant : simulink/Logic and Bit Operations/Compare To Constant  relop===  const=2  OutDataTypeStr=boolean
  Constant1 : Constant  OutDataTypeStr=boolean
  Constant3 : Constant  OutDataTypeStr=boolean
  Data Store Read : DataStoreRead  DataStoreName=VCU_Mode
  Data Store Read3 : DataStoreRead  DataStoreName=SPI3_CS
  LS_EN1 : mbd_mpc574x_ec_toolbox/GPIO Blocks/Digital_Output  Priority=1  gpio_pin=PTF10: [SIUL2_GPIO90 | General Purpose IO PF[10]]  gpio_drive_strength=Disabled
  LS_rst : mbd_mpc574x_ec_toolbox/GPIO Blocks/Digital_Output  Priority=1  gpio_pin=PTC14: [SIUL2_GPIO46 | General Purpose IO PC[14]]  gpio_drive_strength=Disabled
  Logical Operator : Logic  AllPortsSameDT=off  OutDataTypeStr=boolean
  Subsystem : Subsystem
  wires:
  Constant1/1 -> LS_EN1/1
  Constant3/1 -> LS_rst/1
  Data Store Read/1 -> Compare To Constant/1
  Data Store Read3/1 -> Logical Operator/2
  Compare To Constant/1 -> Logical Operator/1
  Logical Operator/1 -> Subsystem/Enable

== system ZT_VehCtrl_18B/VehCtrl/EnergyManage1/Subsystem ==
  VehTrqTgt : Inport
  VehSpd : Inport  Port=2
  MCU_PTO : Inport  Port=3
  Add : Sum
  Bus Selector3 : BusSelector  OutputSignals=MCU2VCU_1.MCU_TrqEst,MCU2VCU_1.MCU_SpdEst
  Constant2 : Constant  Value=WhlRadius
  Constant3 : Constant  Value=9.55  OutDataTypeStr=single
  Divide : Product  Inputs=*/
  Divide1 : Product  Inputs=*/
  Product : Product
  Product1 : Product
  PwrCmd : Outport
  wires:
  Constant3/1 -> Divide1/2
  Divide/1 -> Product/2
  Product/1 -> Add/1
  Constant2/1 -> Divide/2
  Bus Selector3/2 -> Divide1/1  "<MCU_SpdEst>"
  Divide1/1 -> Product1/2
  Product1/1 -> Add/2
  Bus Selector3/1 -> Product1/1  "<MCU_TrqEst>"
  VehTrqTgt/1 -> Product/1
  VehSpd/1 -> Divide/1
  Add/1 -> PwrCmd/1
  MCU_PTO/1 -> Bus Selector3/1

== system ZT_VehCtrl_18B/VehCtrl/FaultProc/Subsystem5 ==
  note: 1-正常
      | 0-超时
  note: 1-丢包
      | 0-正常
  AutoDrive : Inport
  Bus Selector7 : BusSelector  OutputSignals=signal1.AUTO_LiveCnt1,signal1.AUTO_CheckSum1,signal1.PacketLossFlg,signal2.AUTO_LiveCnt2,signal2.AUTO_CheckSum2,signal2.PacketLossFlg,signal3.AUTO_LiveCnt1,signal3.AUTO_CheckSum1,signal3.PacketLossFlg
  Logical Operator : Logic  Operator=NOT  AllPortsSameDT=off  OutDataTypeStr=boolean
  Logical Operator1 : Logic  Operator=OR  Inputs=3  AllPortsSameDT=off  OutDataTypeStr=boolean
  Logical Operator2 : Logic  Inputs=3  AllPortsSameDT=off  OutDataTypeStr=boolean
  PacketLoss_RMT : Stateflow chart  TreatAsAtomicUnit=on
  PacketLoss_RMT1 : Stateflow chart  TreatAsAtomicUnit=on
  PacketLoss_RMT2 : Stateflow chart  TreatAsAtomicUnit=on
  TimeOutLevel_RMT : Stateflow chart  TreatAsAtomicUnit=on
  TimeOutLevel_RMT1 : Stateflow chart  TreatAsAtomicUnit=on
  TimeOutLevel_RMT2 : Stateflow chart  TreatAsAtomicUnit=on
  TimeOut : Outport
  PacketLoss : Outport  Port=2
  wires:
  TimeOutLevel_RMT/1(TimeOutLevel) -> Logical Operator2/1  "TimeOutLevel1"
  Logical Operator2/1 -> Logical Operator/1
  [Auto_LiveCounter] -> TimeOutLevel_RMT/1(LiveCounter)
  Logical Operator1/1 -> PacketLoss/1
  [Auto_PacketLossFlg] -> PacketLoss_RMT/2(PacketLoss)
  [Auto_CheckSumFlg] -> PacketLoss_RMT/1(CheckSum)
  PacketLoss_RMT/1(PacketLossFlg) -> Logical Operator1/1
  AutoDrive/1 -> Bus Selector7/1
  Logical Operator/1 -> TimeOut/1
  [Auto_LiveCounter2] -> TimeOutLevel_RMT1/1(LiveCounter)
  TimeOutLevel_RMT1/1(TimeOutLevel) -> Logical Operator2/2  "TimeOutLevel1"
  [Auto_CheckSumFlg2] -> PacketLoss_RMT1/1(CheckSum)
  [Auto_PacketLossFlg2] -> PacketLoss_RMT1/2(PacketLoss)
  PacketLoss_RMT1/1(PacketLossFlg) -> Logical Operator1/2
  Bus Selector7/6 -> [Auto_PacketLossFlg2]  "<PacketLossFlg>"
  Bus Selector7/5 -> [Auto_CheckSumFlg2]  "<AUTO_CheckSum2>"
  Bus Selector7/4 -> [Auto_LiveCounter2]  "<AUTO_LiveCnt2>"
  Bus Selector7/3 -> [Auto_PacketLossFlg]  "<PacketLossFlg>"
  Bus Selector7/2 -> [Auto_CheckSumFlg]  "<AUTO_CheckSum1>"
  Bus Selector7/1 -> [Auto_LiveCounter]  "<AUTO_LiveCnt1>"
  Bus Selector7/7 -> [Auto_LiveCounter3]  "<AUTO_LiveCnt1>"
  Bus Selector7/8 -> [Auto_CheckSumFlg3]  "<AUTO_CheckSum1>"
  Bus Selector7/9 -> [Auto_PacketLossFlg3]  "<PacketLossFlg>"
  [Auto_LiveCounter3] -> TimeOutLevel_RMT2/1(LiveCounter)
  TimeOutLevel_RMT2/1(TimeOutLevel) -> Logical Operator2/3  "TimeOutLevel1"
  [Auto_PacketLossFlg3] -> PacketLoss_RMT2/2(PacketLoss)
  [Auto_CheckSumFlg3] -> PacketLoss_RMT2/1(CheckSum)
  PacketLoss_RMT2/1(PacketLossFlg) -> Logical Operator1/3

== system ZT_VehCtrl_18B/VehCtrl/MontionControl/DriveControl ==
  EN_COM : Inport
  Ready : Inport  Port=2
  Fault : Inport  Port=3
  CMD : Inport  Port=4
  BMS : Inport  Port=5
  VehSpd : Inport  Port=6
  StrReady : Inport  Port=7
  AUTO : Inport  Port=8
  AUTOMode : Inport  Port=9
  RMT : Inport  Port=10
  DCDC : Inport  Port=11
  Brake : Subsystem
  Bus Creator{1..4} (4 alike) : BusCreator  Inputs=4
  Bus Selector : BusSelector  OutputSignals=RMT.RMT1.RMT_CmdAccPct,BrkPct,ModeDir,ModeStr,StrAng,RMT.RMT4.ModeSafety
  Constant : Constant  Value=0  OutDataTypeStr=uint8
  Constant1 : Constant
  Constant2 : Constant  Value=0  OutDataTypeStr=uint8
  Constant3 : Constant  OutDataTypeStr=boolean
  DriveModeTrans : Stateflow chart  TreatAsAtomicUnit=on
  Equal : RelationalOperator  Operator===  OutDataTypeStr=boolean  RndMeth=Simplest
  Logical Operator : Logic  AllPortsSameDT=off  OutDataTypeStr=boolean
  Motor : Subsystem
  MCUFL_OUT : Outport
  MCUFR_OUT : Outport  Port=2
  MCURL_OUT : Outport  Port=3
  MCURR_OUT : Outport  Port=4
  BrkPrsTgt : Outport  Port=5
  EpbSt : Outport  Port=6
  VehTrqTgt : Outport  Port=7
  wires:
  CMD/1 -> Bus Selector/1
  Bus Selector/3 -> DriveModeTrans/5(ModeDirection)  "<ModeDir>"
  Bus Selector/2 -> DriveModeTrans/2(CmdBrk)  "<BrkPct>"
  Brake/1(BrkPrsTgt) -> BrkPrsTgt/1
  DriveModeTrans/1(VehBrk) -> Brake/1(VehBrkTgt)
  DriveModeTrans/2(EpbSt) -> EpbSt/1
  VehSpd/1 -> DriveModeTrans/9(VehSpd), Motor/5(VehSpd)
  DriveModeTrans/3(VehDrv) -> Motor/1(VehDrvPct)
  Bus Selector/1 -> DriveModeTrans/1(CmdDrv)  "<RMT_CmdAccPct>"
  Bus Selector/4 -> Logical Operator/1  "<ModeStr>"
  StrReady/1 -> DriveModeTrans/8(StrReady)
  DriveModeTrans/4(SpdTgt) -> Motor/2(CmdSpd)
  DriveModeTrans/5(ModeSpd) -> Motor/3(ModeSpeed)
  DriveModeTrans/6(DrvPhase) -> Motor/4(DrvPhase)
  Bus Selector/5 -> Motor/6(CmdStrAng)  "<StrAng>"
  Motor/2(MtrDirCmdFL) -> Bus Creator1/2  "DirCmd"
  Motor/1(Enable) -> Bus Creator1/1, Bus Creator2/1, Bus Creator4/1, Bus Creator3/1  "Enable"
  Bus Creator4/1 -> MCURR_OUT/1
  Bus Creator2/1 -> MCUFR_OUT/1
  Motor/13(MtrSpdCmdRR) -> Bus Creator4/4  "SpdCmd"
  Motor/12(MtrTrqCmdRR) -> Bus Creator4/3  "TrqCmd"
  Motor/11(MtrDirCmdRR) -> Bus Creator4/2  "DirCmd"
  Bus Creator1/1 -> MCUFL_OUT/1
  Motor/7(MtrSpdCmdFR) -> Bus Creator2/4  "SpdCmd"
  Motor/6(MtrTrqCmdFR) -> Bus Creator2/3  "TrqCmd"
  Bus Creator3/1 -> MCURL_OUT/1
  Motor/10(MtrSpdCmdRL) -> Bus Creator3/4  "SpdCmd"
  Motor/4(MtrSpdCmdFL) -> Bus Creator1/4  "SpdCmd"
  Motor/9(MtrTrqCmdRL) -> Bus Creator3/3  "TrqCmd"
  Motor/3(MtrTrqCmdFL) -> Bus Creator1/3  "TrqCmd"
  Motor/8(MtrDirCmdRL) -> Bus Creator3/2  "DirCmd"
  Motor/5(MtrDirCmdFR) -> Bus Creator2/2  "DirCmd"
  Ready/1 -> Motor/9(Ready)
  Motor/14(VehTrqTgt) -> VehTrqTgt/1
  Constant/1 -> DriveModeTrans/3(ModeDrive)
  Constant1/1 -> DriveModeTrans/4(CmdPark)
  Constant2/1 -> DriveModeTrans/7(CmdSpd)
  Bus Selector/6 -> Equal/1, Motor/7(ModeSafety)  "<ModeSafety>"
  AUTO/1 -> Motor/10(AUTO)
  AUTOMode/1 -> Motor/11(AUTOMode)
  BMS/1 -> Motor/12(BMS)
  RMT/1 -> Motor/13(RMT)
  DCDC/1 -> Motor/14(DCDC)
  Fault/1 -> Brake/2(In2), Motor/8(Fault)
  Logical Operator/1 -> DriveModeTrans/6(ModeSteer)
  Equal/1 -> Logical Operator/2
  Constant3/1 -> Equal/2
  EN_COM/1 -> Motor/15(EN_COM)

== system ZT_VehCtrl_18B/VehCtrl/MontionControl/PtoControl ==
  CMD : Inport
  Fault : Inport  Port=2
  Ready : Inport  Port=3
  AUTOMode : Inport  Port=4
  AUTO : Inport  Port=5
  Bus Creator : BusCreator  Inputs=4
  Bus Selector : BusSelector  OutputSignals=ShutDown,NonDrive,NonPto
  Bus Selector1 : BusSelector  OutputSignals=RMT.RMT4.RMT_PtoMode
  Bus Selector2 : BusSelector  OutputSignals=signal2.AUTO_PtoSpd
  Constant5 : Constant  Value=0  OutDataTypeStr=single
  Constant6 : Constant  OutDataTypeStr=uint8
  Constant7 : Constant  Value=0  OutDataTypeStr=uint8
  Logical Operator : Logic  Operator=OR  Inputs=3  AllPortsSameDT=off  OutDataTypeStr=boolean
  Logical Operator1 : Logic  AllPortsSameDT=off  OutDataTypeStr=boolean
  NOT : Logic  Operator=NOT  IconShape=distinctive  AllPortsSameDT=off  OutDataTypeStr=boolean
  Subsystem : Subsystem
  Subsystem1 : Subsystem
  Switch2 : Switch  Criteria=u2 > Threshold
  MCU_PTO_OUT : Outport
  wires:
  CMD/1 -> Bus Selector1/1
  Constant5/1 -> Bus Creator/3  "MtrTrqCmd"
  Subsystem/1(ModeReq) -> Bus Creator/1  "ModeReq"
  Constant6/1 -> Subsystem/1(ModeSpeed)
  Constant7/1 -> Subsystem/2(DirCmd)
  Fault/1 -> Bus Selector/1
  Bus Selector/1 -> Logical Operator/1  "<ShutDown>"
  Bus Selector/2 -> Logical Operator/2  "<NonDrive>"
  Bus Selector/3 -> Logical Operator/3  "<NonPto>"
  Logical Operator/1 -> NOT/1
  Ready/1 -> Logical Operator1/2
  NOT/1 -> Logical Operator1/1
  Logical Operator1/1 -> Bus Creator/4  "Enable"
  Bus Creator/1 -> MCU_PTO_OUT/1
  AUTOMode/1 -> Switch2/2
  Bus Selector1/1 -> Subsystem1/1(<RMT_PtoMode>)  "<RMT_PtoMode>"
  AUTO/1 -> Bus Selector2/1
  Bus Selector2/1 -> Switch2/1  "<AUTO_PtoSpd>"
  Switch2/1 -> Bus Creator/2  "MtrSpdCmd"
  Subsystem1/1(MtrSpdCmd) -> Switch2/3

== system ZT_VehCtrl_18B/VehCtrl/MontionControl/SteerControl ==
  note: 这个是模式，不是方向
  VehSpd : Inport
  CMD : Inport  Port=2
  BDX : Inport  Port=3
  Bus Selector : BusSelector  OutputSignals=ModeStr,StrAng
  Bus Selector1 : BusSelector  OutputSignals=AVCU.BDX_SteeringAngle
  Chart : Stateflow chart  TreatAsAtomicUnit=on
  Constant2 : Constant  Value=10  OutDataTypeStr=uint8
  GreaterThan : RelationalOperator  Operator=<  OutDataTypeStr=boolean  RndMeth=Simplest
  StrReady : Outport
  AngCmd : Outport  Port=2
  wires:
  CMD/1 -> Bus Selector/1
  Bus Selector/1 -> Chart/2(Mode)  "<ModeStr>"
  Bus Selector/2 -> Chart/3(AngCmd)  "<StrAng>"
  BDX/1 -> Bus Selector1/1
  Bus Selector1/1 -> Chart/4(Ang)  "<BDX_SteeringAngle>"
  Chart/2(StrPhase) -> GreaterThan/1
  GreaterThan/1 -> StrReady/1
  Constant2/1 -> GreaterThan/2
  VehSpd/1 -> Chart/1(VehSpd)
  Chart/1(AngCmdOut) -> AngCmd/1

== system ZT_VehCtrl_18B/VehCtrl/MontionControl/ValveControl ==
  note: 仅在安全模式下才能控制
  BrkPrsTgt : Inport
  EpbSt : Inport  Port=2
  BDX : Inport  Port=3
  CMD : Inport  Port=4
  Ready : Inport  Port=5
  "AngCmd " : Inport  Port=6
  fault : Inport  Port=7
  VehSpd : Inport  Port=8
  BrakeSys : Subsystem
  Bus Creator : BusCreator  Inputs=9
  Bus Selector : BusSelector  OutputSignals=ModeSusp,RMT.RMT4.ModeSafety,RMT.RMT2.RMT_ModeWidth
  Bus Selector1 : BusSelector  OutputSignals=AVCU.BDX_BrakePressure
  Bus Selector2 : BusSelector  OutputSignals=NonDrive
  EpbSys : Subsystem
  PumpSys : Subsystem
  SteerSys : Subsystem
  SuspesionSys : Subsystem
  WidthSys : Subsystem
  BDX_OUT : Outport
  wires:
  CMD/1 -> Bus Selector/1
  BDX/1 -> Bus Selector1/1
  BrkPrsTgt/1 -> BrakeSys/1(BrkPrsTgt)
  Bus Selector1/1 -> BrakeSys/2(BrkPrs)  "<BDX_BrakePressure>"
  Bus Selector/1 -> SuspesionSys/1(SuspSt)  "<ModeSusp>"
  Bus Selector/3 -> WidthSys/2(<RMT_ModeWidth>)  "<RMT_ModeWidth>"
  BrakeSys/1(BrkValve) -> Bus Creator/2  "BrkValve"
  SuspesionSys/1(SuspUpValve) -> Bus Creator/6  "SuspUpValve"
  PumpSys/1(Pump) -> Bus Creator/1  "Pump"
  EpbSys/1(EpbValve) -> Bus Creator/5  "EpbValve"
  SteerSys/1(SteerValveL) -> Bus Creator/3  "SteerValveL"
  WidthSys/1(WidthLengthenValve) -> Bus Creator/8  "WidthLengthenValve"
  WidthSys/2(WidthShortenValve) -> Bus Creator/9  "WidthShortenValve"
  Bus Creator/1 -> BDX_OUT/1
  SteerSys/2(SteerValveR) -> Bus Creator/4  "SteerValveR"
  EpbSt/1 -> EpbSys/1(EpbSt)
  SuspesionSys/2(SuspDownValve) -> Bus Creator/7  "SuspDownValve"
  Ready/1 -> PumpSys/1(Ready)
  Bus Selector/2 -> WidthSys/1(ModeSafety), SuspesionSys/2(ModeSafety)  "<ModeSafety>"
  fault/1 -> Bus Selector2/1
  Bus Selector2/1 -> SteerSys/2(In2)  "<NonDrive>"
  VehSpd/1 -> SteerSys/3(VehSpd)
  "AngCmd "/1 -> SteerSys/1(AngCmd)

== system ZT_VehCtrl_18B/VehCtrl/TempertureControl/Lv_to_Dut1 ==
  note: 就是整型，不要替换为single
  MCUReqMtrPumpLv : Inport
  2-D Lookup Table1 : Lookup_n-D  NumberOfTableDimensions=1  BreakpointsForDimension1=uint8([ 0 1 2 3 4 ])  BreakpointsForDimension2=KaTLS_v_DrgUp_X_VehSpd  Table=uint16([ 5 30 40 55 70])  TableDataTypeStr=uint16  ExtrapMethod=Clip  UseLastTableValue=on  OutDataTypeStr=Inherit: Inherit from 'Table data'  RndMeth=Simplest
  Gain : Gain  Gain=1/100  OutDataTypeStr=single
  MCUReqMtrPumpDut : Outport
  wires:
  MCUReqMtrPumpLv/1 -> 2-D Lookup Table1/1
  2-D Lookup Table1/1 -> Gain/1
  Gain/1 -> MCUReqMtrPumpDut/1

== system ZT_VehCtrl_18B/VehCtrl/TempertureControl/Lv_to_Dut2 ==
  note: 就是整型，不要替换为single
  MCUReqMtrPumpLv : Inport
  2-D Lookup Table1 : Lookup_n-D  NumberOfTableDimensions=1  BreakpointsForDimension1=uint8([ 0 1 2 3 4 ])  BreakpointsForDimension2=KaTLS_v_DrgUp_X_VehSpd  Table=uint16([ 5 30 40 55 70])  TableDataTypeStr=uint16  ExtrapMethod=Clip  UseLastTableValue=on  OutDataTypeStr=Inherit: Inherit from 'Table data'  RndMeth=Simplest
  Gain : Gain  Gain=1/100  OutDataTypeStr=single
  MCUReqMtrPumpDut : Outport
  wires:
  MCUReqMtrPumpLv/1 -> 2-D Lookup Table1/1
  2-D Lookup Table1/1 -> Gain/1
  Gain/1 -> MCUReqMtrPumpDut/1

== system ZT_VehCtrl_18B/VehCtrl/TempertureControl/Lv_to_Dut3 ==
  note: 就是整型，不要替换为single
  MCUReqBatPumpLv : Inport
  2-D Lookup Table1 : Lookup_n-D  NumberOfTableDimensions=1  BreakpointsForDimension1=uint8([ 0 1 2 3 4 ])  BreakpointsForDimension2=KaTLS_v_DrgUp_X_VehSpd  Table=uint16([ 5 30 40 55 70])  TableDataTypeStr=uint16  ExtrapMethod=Clip  UseLastTableValue=on  OutDataTypeStr=Inherit: Inherit from 'Table data'  RndMeth=Simplest
  Gain : Gain  Gain=1/100  OutDataTypeStr=single
  MCUReqBatPumpDut : Outport
  wires:
  MCUReqBatPumpLv/1 -> 2-D Lookup Table1/1
  2-D Lookup Table1/1 -> Gain/1
  Gain/1 -> MCUReqBatPumpDut/1

== system ZT_VehCtrl_18B/VehCtrl/TempertureControl/ThermFR_RRvRead1 ==
  RdySt : Inport
  MtrTemp : Inport  Port=2
  Cnt_To_s : Subsystem
  Constant10 : Constant  Value=KeFTM_TK_Way1CoolLv3OnMtrTemp
  Constant11 : Constant  Value=KeFTM_TK_Way1CoolLv2OffMtrTemp
  Constant12 : Constant  Value=KeFTM_TK_Way1CoolLv2OnMtrTemp
  Constant13 : Constant  Value=KeFTM_TK_Way1CoolLv4OnMtrTemp
  Constant7 : Constant  Value=KeFTM_s_Way1OffDlyTime
  Constant8 : Constant  Value=KeFTM_TK_Way1CoolLv4OffMtrTemp
  Constant9 : Constant  Value=KeFTM_TK_Way1CoolLv3OffMtrTemp
  Way1_Cool_Level : Stateflow chart  TreatAsAtomicUnit=on
  MtrPumpLvReq : Outport
  Fan_Low : Outport  Port=2
  wires:
  Way1_Cool_Level/2(MtrPumpLv) -> MtrPumpLvReq/1  "MtrPumpLvReq2"
  Way1_Cool_Level/1(Fan_Low) -> Fan_Low/1  "FanLvReq2"
  RdySt/1 -> Way1_Cool_Level/1(RdySt)
  Constant13/1 -> Way1_Cool_Level/8(Ke_Lv4OnTemp)
  Constant12/1 -> Way1_Cool_Level/4(Ke_Lv2OnTemp)
  Constant10/1 -> Way1_Cool_Level/6(Ke_Lv3OnTemp)
  Constant9/1 -> Way1_Cool_Level/5(Ke_Lv3OffTemp)
  Constant11/1 -> Way1_Cool_Level/3(Ke_Lv2OffTemp)
  Constant7/1 -> Cnt_To_s/1(In1)
  Constant8/1 -> Way1_Cool_Level/7(Ke_Lv4OffTemp)
  Cnt_To_s/1(Out1) -> Way1_Cool_Level/9(Ke_OffDlyCnt)
  MtrTemp/1 -> Way1_Cool_Level/2(Temp)

== system ZT_VehCtrl_18B/VehCtrl/TempertureControl/ThermFR_RRvRead2 ==
  RdySt : Inport
  MtrTemp : Inport  Port=2
  Cnt_To_s : Subsystem
  Constant10 : Constant  Value=KeFTM_TK_Way1CoolLv3OnMtrTemp
  Constant11 : Constant  Value=KeFTM_TK_Way1CoolLv2OffMtrTemp
  Constant12 : Constant  Value=KeFTM_TK_Way1CoolLv2OnMtrTemp
  Constant13 : Constant  Value=KeFTM_TK_Way1CoolLv4OnMtrTemp
  Constant7 : Constant  Value=KeFTM_s_Way1OffDlyTime
  Constant8 : Constant  Value=KeFTM_TK_Way1CoolLv4OffMtrTemp
  Constant9 : Constant  Value=KeFTM_TK_Way1CoolLv3OffMtrTemp
  Way1_Cool_Level : Stateflow chart  TreatAsAtomicUnit=on
  MtrPumpLvReq : Outport
  Fan_Low : Outport  Port=2
  wires:
  MtrTemp/1 -> Way1_Cool_Level/2(Temp)
  Cnt_To_s/1(Out1) -> Way1_Cool_Level/9(Ke_OffDlyCnt)
  Constant8/1 -> Way1_Cool_Level/7(Ke_Lv4OffTemp)
  Constant7/1 -> Cnt_To_s/1(In1)
  Constant11/1 -> Way1_Cool_Level/3(Ke_Lv2OffTemp)
  Constant9/1 -> Way1_Cool_Level/5(Ke_Lv3OffTemp)
  Constant10/1 -> Way1_Cool_Level/6(Ke_Lv3OnTemp)
  Constant12/1 -> Way1_Cool_Level/4(Ke_Lv2OnTemp)
  Constant13/1 -> Way1_Cool_Level/8(Ke_Lv4OnTemp)
  RdySt/1 -> Way1_Cool_Level/1(RdySt)
  Way1_Cool_Level/1(Fan_Low) -> Fan_Low/1  "FanLvReq2"
  Way1_Cool_Level/2(MtrPumpLv) -> MtrPumpLvReq/1  "MtrPumpLvReq2"
